simulink model "advdyn_model"  (R2021a)
settings: Solver=FixedStepAuto  StartTime=0.0  StopTime=14.0  FixedStep=0.02  RelTol=1e-3
values from neighbouring files (symbols this model uses):
  lambda1 = (I2-I3)/I1    (= 1.05426829268)    [EulerEqsSolved.m]    (also in advdyn.m = 0.215769042325)
  lambda2 = (I3-I1)/I2    (= -0.821081081081)    [EulerEqsSolved.m]    (also in advdyn.m = -0.97926125905)
  lambda3 = (I1-I2)/I3    (= -1.73553719008)    [EulerEqsSolved.m]    (also in advdyn.m = 0.96803177906)
  omega0 = [0.001, 0.001, 10]    [advdyn.m]
settings Model: Creator=matthewearl  LastModifiedBy=matthewearl

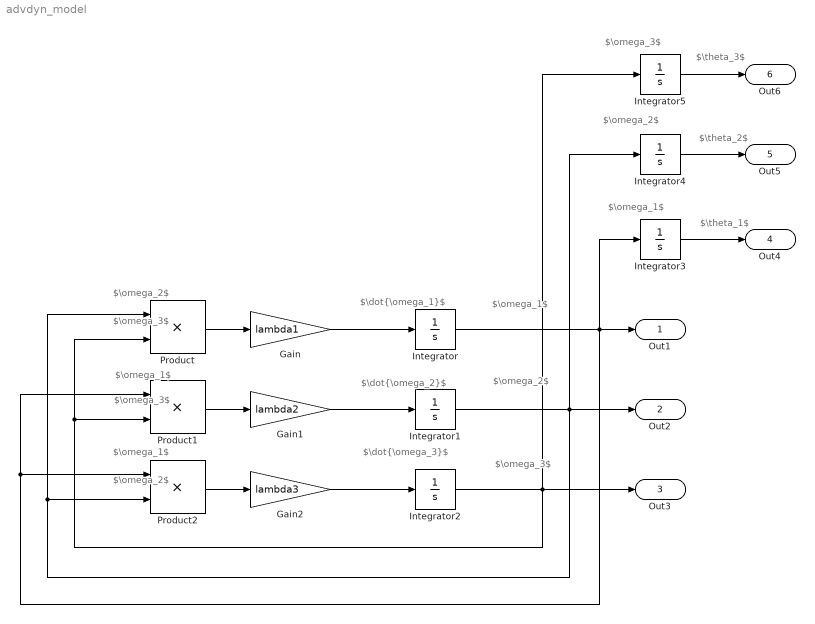
== system advdyn_model ==
  note: $\dot{\omega_1}$
  note: $\dot{\omega_2}$
  note: $\dot{\omega_3}$
  note: $\omega_1$
  note: $\omega_2$
  note: $\omega_3$
  note: $\omega_1$
  note: $\omega_1$
  note: $\omega_2$
  note: $\omega_2$
  note: $\omega_3$
  note: $\omega_3$
  note: $\omega_1$
  note: $\omega_2$
  note: $\omega_3$
  note: $\theta_1$
  note: $\theta_2$
  note: $\theta_3$
  Gain : Gain  Gain=lambda1
  Gain1 : Gain  Gain=lambda2
  Gain2 : Gain  Gain=lambda3
  Integrator : Integrator  InitialCondition=omega0(1)
  Integrator1 : Integrator  InitialCondition=omega0(2)
  Integrator2 : Integrator  InitialCondition=omega0(3)
  Integrator3 : Integrator
  Integrator4 : Integrator
  Integrator5 : Integrator
  Product : Product
  Product1 : Product
  Product2 : Product
  Out1 : Outport  SignalName=omega1
  Out2 : Outport  Port=2  SignalName=omega2
  Out3 : Outport  Port=3  SignalName=omega3
  Out4 : Outport  Port=4  SignalName=theta1
  Out5 : Outport  Port=5  SignalName=theta2
  Out6 : Outport  Port=6  SignalName=theta3
  wires:
  Product2/1 -> Gain2/1
  Product1/1 -> Gain1/1
  Product/1 -> Gain/1
  Gain/1 -> Integrator/1
  Gain2/1 -> Integrator2/1
  Gain1/1 -> Integrator1/1
  Integrator2/1 -> Integrator5/1, Out3/1, Product/2, Product1/2
  Integrator1/1 -> Integrator4/1, Out2/1, Product/1, Product2/2
  Integrator/1 -> Integrator3/1, Out1/1, Product1/1, Product2/1
  Integrator3/1 -> Out4/1
  Integrator4/1 -> Out5/1
  Integrator5/1 -> Out6/1
